simulink model "attitudeKalman"  (R2020b)
settings: Solver=VariableStepAuto  StartTime=0.0  StopTime=60  RelTol=1e-3
values from neighbouring files (symbols this model uses):
  Bw0 = [10;-20;-30]*pi/180    [main.m]
  Bwhat0 = [0;0;0]    [main.m]
  dt_gyros = 0.01    [main.m]
  dt_sim = 0.001    [main.m]
  dt_v1 = 1    [main.m]
  dt_v2 = 10    [main.m]
  nb_seed = randi([0, 2^32], 3, 1)    [main.m]
  nv1_seed = randi([0, 2^32], 3, 1)    [main.m]
  nv2_seed = randi([0, 2^32], 3, 1)    [main.m]
  nw_seed = randi([0, 2^32], 3, 1)    [main.m]
  P0 = diag([sigmaangle, sigmaangle, sigmaangle,             sigmaomega, sigmaomega, sigmaomega])    [main.m]
  q0_BI = e2q(e, th)    [main.m]
  qhat0_BI = A2q(Ahat0_BI)    [main.m]
  sigmab = 0.1*pi/180    (= 0.00174532925199)    [main.m]
  sigmav1 = 1*pi/180    (= 0.0174532925199)    [main.m]
  sigmav2 = 0.1*pi/180    (= 0.00174532925199)    [main.m]
  sigmaw = 1*pi/180    (= 0.0174532925199)    [main.m]
  v1_I = [1;0;0]    [main.m]
  v2_I = [0;1;0]    [main.m]
  wbi0_B = [-10; 20; -30]*pi/180    [main.m]
undefined symbols (not defined in the file or in its folder): J_C_B
libraries: simulink x3
settings Model: Creator=tjones  LastModifiedBy=tjones

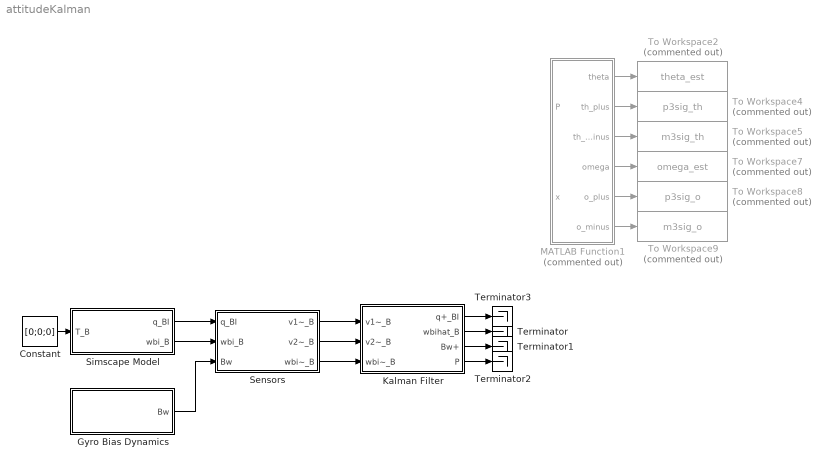
== system attitudeKalman ==
  Constant : Constant  Value=[0;0;0]
  Gyro Bias Dynamics : Subsystem
  Kalman Filter : Subsystem
  MATLAB Function1 : MATLAB Function  Commented=on  TreatAsAtomicUnit=on
  Sensors : Subsystem
  Simscape Model : Subsystem  TreatAsAtomicUnit=on
  Terminator{,1..3} (4 alike) : Terminator
  To Workspace2 : ToWorkspace  Commented=on  VariableName=theta_est  SaveFormat=Timeseries  SampleTime=-1
  To Workspace4 : ToWorkspace  Commented=on  VariableName=p3sig_th  SaveFormat=Timeseries  SampleTime=-1
  To Workspace5 : ToWorkspace  Commented=on  VariableName=m3sig_th  SaveFormat=Timeseries  SampleTime=-1
  To Workspace7 : ToWorkspace  Commented=on  VariableName=omega_est  SaveFormat=Timeseries  SampleTime=-1
  To Workspace8 : ToWorkspace  Commented=on  VariableName=p3sig_o  SaveFormat=Timeseries  SampleTime=-1
  To Workspace9 : ToWorkspace  Commented=on  VariableName=m3sig_o  SaveFormat=Timeseries  SampleTime=-1
  wires:
  MATLAB Function1/1(theta) -> To Workspace2/1
  MATLAB Function1/2(th_plus) -> To Workspace4/1
  MATLAB Function1/3(th_minus) -> To Workspace5/1
  MATLAB Function1/4(omega) -> To Workspace7/1
  MATLAB Function1/5(o_plus) -> To Workspace8/1
  MATLAB Function1/6(o_minus) -> To Workspace9/1
  Constant/1 -> Simscape Model/1(T_B)
  Simscape Model/1(q_BI) -> Sensors/1(q_BI)
  Simscape Model/2(wbi_B) -> Sensors/2(wbi_B)
  Gyro Bias Dynamics/1(Bw) -> Sensors/3(Bw)
  Sensors/1(v1~_B) -> Kalman Filter/1(v1~_B)
  Sensors/2(v2~_B) -> Kalman Filter/2(v2~_B)
  Sensors/3(wbi~_B) -> Kalman Filter/3(wbi~_B)
  Kalman Filter/4(P) -> Terminator2/1
  Kalman Filter/1(q+_BI) -> Terminator3/1
  Kalman Filter/2(wbihat_B) -> Terminator/1
  Kalman Filter/3(Bw+) -> Terminator1/1

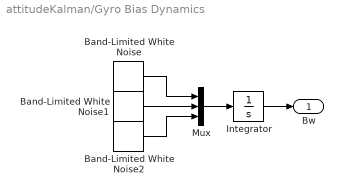
== system attitudeKalman/Gyro Bias Dynamics ==
  Band-Limited White Noise : simulink/Sources/Band-Limited White Noise  Cov=[sigmab^2]  Ts=dt_sim  seed=[nb_seed(1)]
  Band-Limited White Noise1 : simulink/Sources/Band-Limited White Noise  Cov=[sigmab^2]  Ts=dt_sim  seed=[nb_seed(2)]
  Band-Limited White Noise2 : simulink/Sources/Band-Limited White Noise  Cov=[sigmab^2]  Ts=dt_sim  seed=[nb_seed(3)]
  Integrator : Integrator  InitialCondition=Bw0
  Mux : Mux  Inputs=3
  Bw : Outport
  wires:
  Integrator/1 -> Bw/1
  Band-Limited White Noise1/1 -> Mux/2
  Band-Limited White Noise/1 -> Mux/1
  Band-Limited White Noise2/1 -> Mux/3
  Mux/1 -> Integrator/1

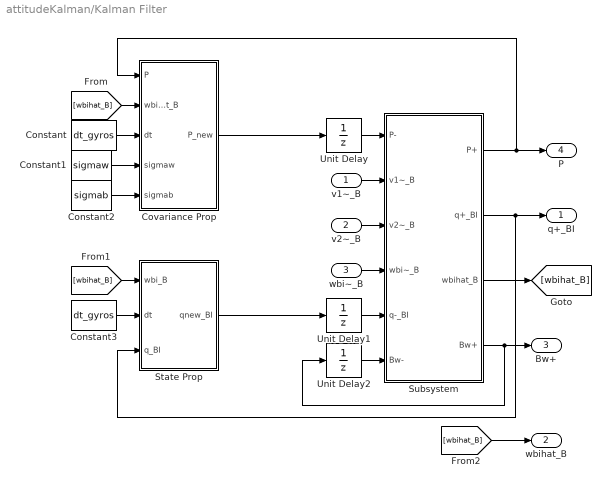
== system attitudeKalman/Kalman Filter ==
  v1~_B : Inport
  v2~_B : Inport  Port=2
  wbi~_B : Inport  Port=3
  Constant : Constant  Value=dt_gyros
  Constant1 : Constant  Value=sigmaw
  Constant2 : Constant  Value=sigmab
  Constant3 : Constant  Value=dt_gyros
  Covariance Prop : MATLAB Function  TreatAsAtomicUnit=on
  State Prop : MATLAB Function  TreatAsAtomicUnit=on
  Subsystem : Subsystem
  Unit Delay : UnitDelay  InitialCondition=P0  SampleTime=dt_gyros  HasFrameUpgradeWarning=on
  Unit Delay1 : UnitDelay  InitialCondition=qhat0_BI  SampleTime=dt_gyros  HasFrameUpgradeWarning=on
  Unit Delay2 : UnitDelay  InitialCondition=Bwhat0  SampleTime=dt_gyros  HasFrameUpgradeWarning=on
  q+_BI : Outport  OutDataTypeStr=Bus: qBus
  wbihat_B : Outport  Port=2
  Bw+ : Outport  Port=3
  P : Outport  Port=4
  wires:
  Covariance Prop/1(P_new) -> Unit Delay/1
  State Prop/1(qnew_BI) -> Unit Delay1/1
  Subsystem/2(q+_BI) -> State Prop/3(q_BI), q+_BI/1
  Subsystem/1(P+) -> P/1, Covariance Prop/1(P)
  Unit Delay/1 -> Subsystem/1(P-)
  Subsystem/4(Bw+) -> Unit Delay2/1, Bw+/1
  Subsystem/3(wbihat_B) -> [wbihat_B]
  [wbihat_B] -> Covariance Prop/2(wbihat_B)
  Constant/1 -> Covariance Prop/3(dt)
  Constant1/1 -> Covariance Prop/4(sigmaw)
  Constant2/1 -> Covariance Prop/5(sigmab)
  [wbihat_B] -> State Prop/1(wbi_B)
  Constant3/1 -> State Prop/2(dt)
  Unit Delay2/1 -> Subsystem/6(Bw-)
  Unit Delay1/1 -> Subsystem/5(q-_BI)
  wbi~_B/1 -> Subsystem/4(wbi~_B)
  v2~_B/1 -> Subsystem/3(v2~_B)
  v1~_B/1 -> Subsystem/2(v1~_B)
  [wbihat_B] -> wbihat_B/1

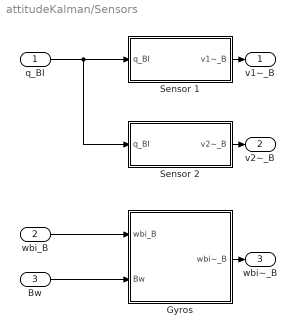
== system attitudeKalman/Sensors ==
  q_BI : Inport  OutDataTypeStr=Bus: qBus
  wbi_B : Inport  Port=2
  Bw : Inport  Port=3
  Gyros : Subsystem
  Sensor 1 : Subsystem
  Sensor 2 : Subsystem
  v1~_B : Outport
  v2~_B : Outport  Port=2
  wbi~_B : Outport  Port=3
  wires:
  Sensor 1/1(v1~_B) -> v1~_B/1
  Sensor 2/1(v2~_B) -> v2~_B/1
  q_BI/1 -> Sensor 2/1(q_BI), Sensor 1/1(q_BI)
  Gyros/1(wbi~_B) -> wbi~_B/1
  Bw/1 -> Gyros/2(Bw)
  wbi_B/1 -> Gyros/1(wbi_B)

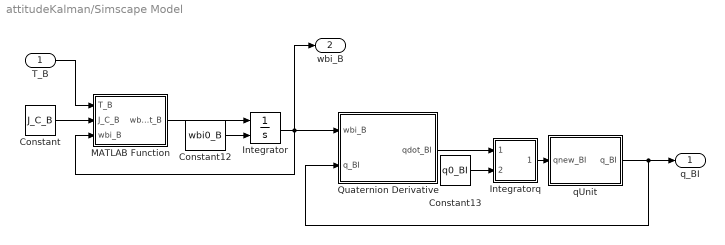
== system attitudeKalman/Simscape Model ==
  T_B : Inport
  Constant : Constant  Value=J_C_B
  Constant12 : Constant  Value=wbi0_B
  Constant13 : Constant  Value=q0_BI  OutDataTypeStr=Bus: qBus
  Integrator : Integrator  InitialConditionSource=external
  Integratorq : Subsystem
  MATLAB Function : MATLAB Function  TreatAsAtomicUnit=on
  Quaternion Derivative : MATLAB Function  TreatAsAtomicUnit=on
  qUnit : MATLAB Function  TreatAsAtomicUnit=on
  q_BI : Outport  OutDataTypeStr=Bus: qBus  VectorParamsAs1DForOutWhenUnconnected=off
  wbi_B : Outport  Port=2  VectorParamsAs1DForOutWhenUnconnected=off
  wires:
  qUnit/1(q_BI) -> q_BI/1, Quaternion Derivative/2(q_BI)
  Integratorq/1(qnew_BI) -> qUnit/1(qnew_BI)
  Quaternion Derivative/1(qdot_BI) -> Integratorq/1(qdot_BI)
  Constant13/1 -> Integratorq/2(q0_BI)
  MATLAB Function/1(wbidot_B) -> Integrator/1
  Constant12/1 -> Integrator/2
  Constant/1 -> MATLAB Function/2(J_C_B)
  Integrator/1 -> wbi_B/1, MATLAB Function/3(wbi_B), Quaternion Derivative/1(wbi_B)
  T_B/1 -> MATLAB Function/1(T_B)

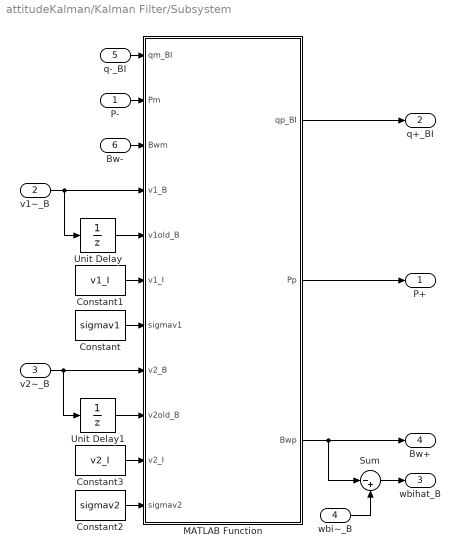
== system attitudeKalman/Kalman Filter/Subsystem ==
  P- : Inport
  v1~_B : Inport  Port=2
  v2~_B : Inport  Port=3
  wbi~_B : Inport  Port=4
  q-_BI : Inport  Port=5  OutDataTypeStr=Bus: qBus
  Bw- : Inport  Port=6
  Constant : Constant  Value=sigmav1  SampleTime=dt_gyros
  Constant1 : Constant  Value=v1_I  SampleTime=dt_gyros
  Constant2 : Constant  Value=sigmav2  SampleTime=dt_gyros
  Constant3 : Constant  Value=v2_I  SampleTime=dt_gyros
  MATLAB Function : MATLAB Function  TreatAsAtomicUnit=on
  Sum : Sum  Inputs=|-+
  Unit Delay : UnitDelay  SampleTime=-1  HasFrameUpgradeWarning=on
  Unit Delay1 : UnitDelay  SampleTime=-1  HasFrameUpgradeWarning=on
  P+ : Outport
  q+_BI : Outport  Port=2  OutDataTypeStr=Bus: qBus
  wbihat_B : Outport  Port=3
  Bw+ : Outport  Port=4
  wires:
  MATLAB Function/2(Pp) -> P+/1
  MATLAB Function/1(qp_BI) -> q+_BI/1
  MATLAB Function/3(Bwp) -> Sum/1, Bw+/1
  Sum/1 -> wbihat_B/1
  wbi~_B/1 -> Sum/2
  Bw-/1 -> MATLAB Function/3(Bwm)
  P-/1 -> MATLAB Function/2(Pm)
  q-_BI/1 -> MATLAB Function/1(qm_BI)
  v1~_B/1 -> MATLAB Function/4(v1_B), Unit Delay/1
  v2~_B/1 -> Unit Delay1/1, MATLAB Function/8(v2_B)
  Constant/1 -> MATLAB Function/7(sigmav1)
  Constant1/1 -> MATLAB Function/6(v1_I)
  Constant2/1 -> MATLAB Function/11(sigmav2)
  Constant3/1 -> MATLAB Function/10(v2_I)
  Unit Delay/1 -> MATLAB Function/5(v1old_B)
  Unit Delay1/1 -> MATLAB Function/9(v2old_B)

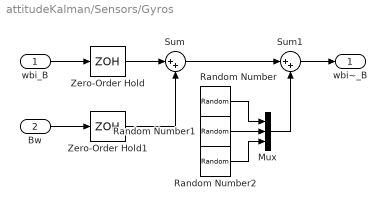
== system attitudeKalman/Sensors/Gyros ==
  wbi_B : Inport
  Bw : Inport  Port=2
  Mux : Mux  Inputs=3
  Random Number : RandomNumber  Variance=[sigmaw^2]  Seed=nw_seed(1)  SampleTime=dt_gyros
  Random Number1 : RandomNumber  Variance=[sigmaw^2]  Seed=nw_seed(2)  SampleTime=dt_gyros
  Random Number2 : RandomNumber  Variance=[sigmaw^2]  Seed=nw_seed(3)  SampleTime=dt_gyros
  Sum : Sum  Inputs=|++
  Sum1 : Sum  Inputs=|++
  Zero-Order Hold : ZeroOrderHold  SampleTime=dt_gyros
  Zero-Order Hold1 : ZeroOrderHold  SampleTime=dt_gyros
  wbi~_B : Outport
  wires:
  wbi_B/1 -> Zero-Order Hold/1
  Bw/1 -> Zero-Order Hold1/1
  Zero-Order Hold/1 -> Sum/1
  Zero-Order Hold1/1 -> Sum/2
  Sum1/1 -> wbi~_B/1
  Sum/1 -> Sum1/1
  Random Number1/1 -> Mux/2
  Random Number/1 -> Mux/1
  Random Number2/1 -> Mux/3
  Mux/1 -> Sum1/2

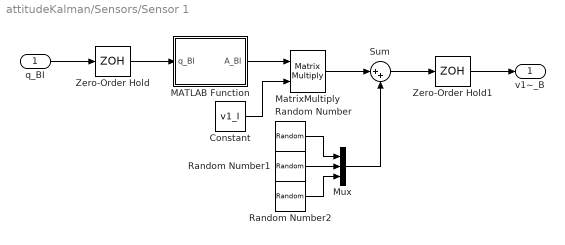
== system attitudeKalman/Sensors/Sensor 1 ==
  q_BI : Inport  OutDataTypeStr=Bus: qBus
  Constant : Constant  Value=v1_I
  MATLAB Function : MATLAB Function  TreatAsAtomicUnit=on
  MatrixMultiply : Product  Multiplication=Matrix(*)
  Mux : Mux  Inputs=3
  Random Number : RandomNumber  Variance=sigmav1^2  Seed=nv1_seed(1)  SampleTime=dt_v1
  Random Number1 : RandomNumber  Variance=sigmav1^2  Seed=nv1_seed(2)  SampleTime=dt_v1
  Random Number2 : RandomNumber  Variance=sigmav1^2  Seed=nv1_seed(3)  SampleTime=dt_v1
  Sum : Sum  Inputs=|++
  Zero-Order Hold : ZeroOrderHold  SampleTime=dt_v1
  Zero-Order Hold1 : ZeroOrderHold  SampleTime=dt_gyros
  v1~_B : Outport
  wires:
  q_BI/1 -> Zero-Order Hold/1
  Zero-Order Hold/1 -> MATLAB Function/1(q_BI)
  MATLAB Function/1(A_BI) -> MatrixMultiply/1
  Constant/1 -> MatrixMultiply/2
  MatrixMultiply/1 -> Sum/1
  Random Number1/1 -> Mux/2
  Random Number/1 -> Mux/1
  Random Number2/1 -> Mux/3
  Mux/1 -> Sum/2
  Zero-Order Hold1/1 -> v1~_B/1
  Sum/1 -> Zero-Order Hold1/1

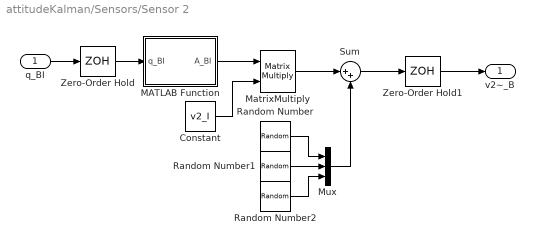
== system attitudeKalman/Sensors/Sensor 2 ==
  q_BI : Inport  OutDataTypeStr=Bus: qBus
  Constant : Constant  Value=v2_I
  MATLAB Function : MATLAB Function  TreatAsAtomicUnit=on
  MatrixMultiply : Product  Multiplication=Matrix(*)
  Mux : Mux  Inputs=3
  Random Number : RandomNumber  Variance=sigmav2^2  Seed=nv2_seed(1)  SampleTime=dt_v2
  Random Number1 : RandomNumber  Variance=sigmav2^2  Seed=nv2_seed(2)  SampleTime=dt_v2
  Random Number2 : RandomNumber  Variance=sigmav2^2  Seed=nv2_seed(3)  SampleTime=dt_v2
  Sum : Sum  Inputs=|++
  Zero-Order Hold : ZeroOrderHold  SampleTime=dt_v2
  Zero-Order Hold1 : ZeroOrderHold  SampleTime=dt_gyros
  v2~_B : Outport
  wires:
  Sum/1 -> Zero-Order Hold1/1
  Zero-Order Hold1/1 -> v2~_B/1
  Mux/1 -> Sum/2
  Random Number2/1 -> Mux/3
  Random Number/1 -> Mux/1
  Random Number1/1 -> Mux/2
  MatrixMultiply/1 -> Sum/1
  Constant/1 -> MatrixMultiply/2
  MATLAB Function/1(A_BI) -> MatrixMultiply/1
  Zero-Order Hold/1 -> MATLAB Function/1(q_BI)
  q_BI/1 -> Zero-Order Hold/1

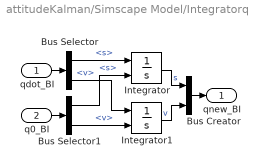
== system attitudeKalman/Simscape Model/Integratorq ==
  qdot_BI : Inport  OutDataTypeStr=Bus: qBus
  q0_BI : Inport  Port=2  OutDataTypeStr=Bus: qBus
  Bus Creator : BusCreator  Inputs=2  OutDataTypeStr=Bus: qBus
      settings: InheritFromInputs=off
  Bus Selector : BusSelector  OutputSignals=s,v
  Bus Selector1 : BusSelector  OutputSignals=s,v
  Integrator : Integrator  InitialConditionSource=external
  Integrator1 : Integrator  InitialConditionSource=external
  qnew_BI : Outport  OutDataTypeStr=Bus: qBus  VectorParamsAs1DForOutWhenUnconnected=off
  wires:
  qdot_BI/1 -> Bus Selector/1
  q0_BI/1 -> Bus Selector1/1
  Bus Selector/1 -> Integrator/1  "<s>"
  Bus Selector1/1 -> Integrator/2  "<s>"
  Bus Selector/2 -> Integrator1/1  "<v>"
  Bus Selector1/2 -> Integrator1/2  "<v>"
  Integrator/1 -> Bus Creator/1  "s"
  Integrator1/1 -> Bus Creator/2  "v"
  Bus Creator/1 -> qnew_BI/1

== matlab function attitudeKalman/Simscape Model/qUnit ==
  data: qnew_BI input Bus: qBus; q_BI output Bus: qBus
function q_BI = fcn(qnew_BI)

q_BI = qUnit(qnew_BI);

== matlab function attitudeKalman/Kalman Filter/Covariance Prop ==
  data: P input; P_new output; wbihat_B input; dt input; sigmaw input; sigmab input
function P_new = fcn(P,wbihat_B,dt,sigmaw,sigmab)

wX = X(wbihat_B);
wmag = norm(wbihat_B);
I3 = eye(3);

% Calculate Phi11 according to Equation 6.83b
Phi11 = I3 - wX*sin(wmag*dt)/wmag + wX*wX*(1-cos(wmag*dt))/wmag^2;
% Calculate Phi12 according to Equation 6.83c
Phi12 = wX*(1-cos(wmag*dt))/wmag^2 - I3*dt - ...
        wX*wX*(wmag*dt-sin(wmag*dt))/wmag^3;

% Equation 6.83a
Phi = [Phi11, Phi12; zeros(3,3), I3];

% Equation 6.93
Qd = [(sigmaw^2*dt + (sigmab^2*dt^3)/3)*I3, -(sigmab^2*dt^2)*I3/2;...
                     -(sigmab^2*dt^2)*I3/2,      (sigmab^2*dt)*I3];

P_new = Phi*P*Phi' + Qd; % from Table 6.3

== matlab function attitudeKalman/Simscape Model/MATLAB Function ==
  data: T_B input; wbidot_B output; J_C_B input; wbi_B input
function wbidot_B = fcn(T_B, J_C_B, wbi_B)

wbidot_B = J_C_B\(T_B - cross(wbi_B, J_C_B*wbi_B));

== matlab function attitudeKalman/Kalman Filter/State Prop ==
  data: wbi_B input; dt input; qnew_BI output Bus: qBus; q_BI input Bus: qBus
function qnew_BI = fcn(wbi_B, dt, q_BI)

w_mag = norm(wbi_B);

psi = sin(1/2*w_mag*dt)*wbi_B/w_mag;

qnew_BI.s = cos(1/2*w_mag*dt)*q_BI.s - psi'*q_BI.v;
qnew_BI.v = psi*q_BI.s + (cos(1/2*w_mag*dt)*eye(3) - X(psi))*q_BI.v;
qnew_BI = qUnit(qnew_BI);

== matlab function attitudeKalman/Kalman Filter/Subsystem/MATLAB Function ==
  data: qm_BI input Bus: qBus; qp_BI output Bus: qBus; Pm input; Bwm input; v1_B input; v1old_B input; v1_I input; sigmav1 input; v2_B input; v2old_B input; v2_I input; sigmav2 input; Pp output; Bwp output
function [qp_BI,Pp,Bwp] = fcn(qm_BI,Pm,Bwm,v1_B,v1old_B,v1_I,sigmav1,v2_B,v2old_B,v2_I,sigmav2)

if v1_B ~= v1old_B
    [qm_BI, Pm, Bwm] = update(qm_BI, Pm, Bwm, v1_B, v1_I, sigmav1);
end

if v2_B ~= v2old_B
    [qp_BI, Pp, Bwp] = update(qm_BI, Pm, Bwm, v2_B, v2_I, sigmav2);
else
    qp_BI = qm_BI;
    Pp = Pm;
    Bwp = Bwm;
    
end

== matlab function attitudeKalman/MATLAB Function1 ==
  data: P input; theta output; x input; th_plus output; th_minus output; omega output; o_plus output; o_minus output
function [theta,th_plus,th_minus,omega,o_plus,o_minus] = fcn(P, x)

theta = x(1);
th_plus = theta + 3*sqrt(P(1,1));
th_minus = theta - 3*sqrt(P(1,1));

omega = x(2);
o_plus = omega + 3*sqrt(P(2,2));
o_minus = omega - 3*sqrt(P(2,2));

== matlab function attitudeKalman/Simscape Model/Quaternion Derivative ==
  data: wbi_B input; q_BI input Bus: qBus; qdot_BI output Bus: qBus
function qdot_BI = fcn(wbi_B, q_BI)

w.s = 0;
w.v = wbi_B;

qdot = qX(w, q_BI);

qdot_BI.s = 1/2*qdot.s;
qdot_BI.v = 1/2*qdot.v;

== matlab function attitudeKalman/Sensors/Sensor 1/MATLAB Function ==
  data: q_BI input Bus: qBus; A_BI output
function A_BI = fcn(q_BI)

A_BI = q2A(q_BI);

== matlab function attitudeKalman/Sensors/Sensor 2/MATLAB Function ==
  data: q_BI input Bus: qBus; A_BI output
function A_BI = fcn(q_BI)

A_BI = q2A(q_BI);
